simulink model "InitSerialCommunication"  (R2017b)
settings: Solver=FixedStepAuto  StartTime=0.0  StopTime=110  FixedStep=0.01  RelTol=1e-3  EnableMultiTasking=on
settings Model: Creator=Fabio  LastModifiedBy=Fabio
settings SolverCC: AutoInsertRateTranBlk=on
settings DataIOCC: LimitDataPoints=on
settings OptimizationCC: LifeSpan=inf
settings DebuggingCC: AllowSymbolicDim=off  SFUnexpectedBacktrackingDiag=warning  SFNoUnconditionalDefaultTransitionDiag=warning  SFExecutionAtInitializationDiag=none
settings CodeAppCC: StateflowObjectComments=on
settings GRTTargetCC: TargetLangStandard=C89/C90 (ANSI)
settings ConfigComp: CovMetricSettings=dw  CovHtmlReporting=on  CovSaveCumulativeToWorkspaceVar=on  CovSaveSingleToWorkspaceVar=on  CovShowResultsExplorer=off  CovExternalEMLEnable=off

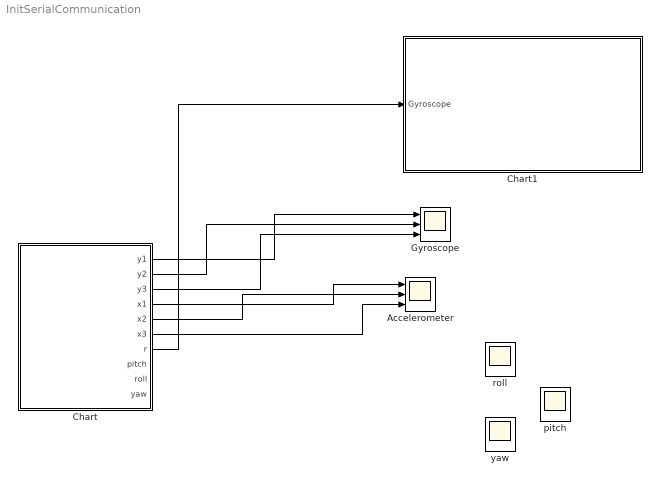
== system InitSerialCommunication ==
  "Accelerometer " : Scope  NumInputPorts=3
  Chart : Stateflow chart  TreatAsAtomicUnit=on
  Chart1 : Stateflow chart  TreatAsAtomicUnit=on
  "Gyroscope " : Scope  NumInputPorts=3
  pitch : Scope
  "roll " : Scope
  yaw : Scope
  wires:
  Chart/1(y1) -> "Gyroscope "/1
  Chart/2(y2) -> "Gyroscope "/2
  Chart/3(y3) -> "Gyroscope "/3
  Chart/4(x1) -> "Accelerometer "/1
  Chart/5(x2) -> "Accelerometer "/2
  Chart/6(x3) -> "Accelerometer "/3
  Chart/7(r) -> Chart1/1(Gyroscope)

== stateflow chart InitSerialCommunication/Chart1 ==
  state AngularPosition
    entry:
    [Ak,qK]=angularPositionEstimation(gyroscope,T,qPrev)
  (default) -> AngularPosition
  data: w function_input; t function_input; q_pre function_input; Ak function_output; qK function_output; Gyroscope input size=3
  function [Ak,qK]=angularPositionEstimation(w,t,q_pre):
    | function [Ak,qK]=angularPositionEstimation(w,t,q_pre)
    | 
    | wx=w(1);
    | wy=w(2);
    | wz=w(3);
    | 
    | 
    | 
    | 
    | 
    | %Calculation of the “a priori” noise covariance matrix
    | 
    | 
    | 
    | end

== stateflow chart InitSerialCommunication/Chart ==
  state Read
    entry:
    [x1,x2,x3,y1,y2,y3,yaw,pitch,roll,r]=readData(connection);
  state Init
    entry:
    connection=initSerialCommunication();
  state Close
    entry: close(connection);
  Read -> Read [order 2]
  (default) -> Init
  Init -> Read
  Read -> Close [order 1] : after(100,sec)
  data: out function_output; accX function_output; accY function_output; accZ function_output; gyroX function_output; gyroY function_output; gyroZ function_output; serialConnection function_input; rotationYaw function_output; rotationPitch function_output; rotationRoll function_output; acc function_output; gyro function_output; rotation function_output; serialConnection function_input; connection local; u local; y1 output; y2 output; y3 output; x1 output; x2 output; x3 output; r output; pitch output; roll output; yaw output
  function out=initSerialCommunication:
    | function out=initSerialCommunication()
    | 
    | 
    |  coder.extrinsic('initSerial');
    |  
    | %Custom some properties before open the serial communication
    | serialPort=initSerial("COM3",9600,64);
    | 
    | 
    | 
    | out=serialPort;
  function [accX,accY,accZ,gyroX,gyroY,gyroZ,rotationYaw,rotationPitch,rotationRoll,acc,gyro,rotation] =readData(serialConnection):
    | function [accX,accY,accZ,gyroX,gyroY,gyroZ,rotationYaw,rotationPitch,rotationRoll,acc,gyro,rotation] =readData(serialConnection)
    | 
    |   coder.extrinsic('read');
    |    
    |   g=9.80664999999998;
    | 
    | 
    |   accX=1;
    |   typecast(accX,'double');
    |   accY=1;
    |   typecast(accY,'double');
    |   accZ=1;
    |   typecast(accZ,'double');
    |   
    |    gyroX=1;
    |   typecast(gyroX,'double');
    |   gyroY=1;
    |   typecast(gyroY,'double');
    |   gyroZ=1;
    |   typecast(gyroZ,'double');
    |   
    |   rotationYaw=1;
    |   typecast(rotationYaw,'double');
    |   rotationPitch=1;
    |   typecast(rotationPitch,'double');
    |   rotationRoll=1;
    |   typecast(rotationRoll,'double');
    | 
    | 
    |   [accX,accY,accZ,gyroX,gyroY,gyroZ,rotationYaw,rotationPitch,rotationRoll]=read(serialConnection);
    |   
    |   accX=accX*g;
    |   accY=accY*g;
    |   accZ=accZ*g;
    | 
    |  acc=[accX,accY,accZ];
    |  gyro=[gyroX,gyroY,gyroZ];
    | 
    | 
    |   rotation=[rotationRoll, rotationPitch, rotationYaw];
  function close(serialConnection):
    | function close(serialConnection)
    |   coder.extrinsic('closeConnection');
    |   
    |   closeConnection(serialConnection);
